simulink model "EV"  (R2023a)
settings: Solver=ode4  StartTime=0.0  StopTime=10  FixedStep=Ts  RelTol=1e-3  EnableMultiTasking=on
PostLoadFcn:
  | Ts=1/1000000;L=1.8e-3;w=2*pi*60;C=20e-6;
InitFcn:
  | Ts=1/1000000;L=1.8e-3;w=2*pi*60;C=20e-6;
undefined symbols (not defined in the file): DiscIntNeverNeededParam
libraries: simulink x13, spsSeriesRLCBranchLib x9, spsIGBTDiodeLib x6, spsGroundLib x5, spsVoltageMeasurementLib x4, spsCurrentMeasurementLib x3, spsDCVoltageSourceLib x1, eePwmGeneratorTwoLevel x1, spspowerguiLib x1
Description:
  | Model of a simple control system for use iin training.
settings Model: Creator=Paul Baracos  LastModifiedBy=Julian
settings SolverCC: AlgebraicLoopSolver=TrustRegion
settings DataIOCC: LimitDataPoints=on  SaveFormat=Array  SignalLoggingSaveFormat=ModelDataLogs  SaveOutput=off  SaveTime=off  ReturnWorkspaceOutputs=off  SignalLoggingName=sigsOut
settings OptimizationCC: BlockReduction=off  BooleanDataType=off  OptimizeBlockIOStorage=off  BufferReuse=off  ReuseModelBlockBuffer=off  GlobalBufferReuse=off  ExpressionFolding=off  LocalBlockOutputs=off  InitFltsAndDblsToZero=on  LifeSpan=inf
settings DebuggingCC: SaveWithParameterizedLinksMsg=none  UnderspecifiedInitializationDetection=Classic  MergeDetectMultiDrivingBlocksExec=none  SignalResolutionControl=TryResolveAllWithWarning  MultiTaskDSMMsg=warning  MultiTaskCondExecSysMsg=none  FcnCallInpInsideContextMsg=warning  UnconnectedInputMsg=warning  UnconnectedOutputMsg=warning  UnconnectedLineMsg=warning  SFUnexpectedBacktrackingDiag=warning  SFNoUnconditionalDefaultTransitionDiag=warning  SFExecutionAtInitializationDiag=none  ArithmeticOperatorsInVariantConditions=warning
settings HardwareCC: ProdBitPerPointer=32  ProdBitPerSizeT=32  ProdBitPerPtrDiffT=32  ProdLargestAtomicFloat=None  ProdIntDivRoundTo=Undefined  ProdEndianess=Unspecified  ProdWordSize=32  ProdHWDeviceType=32-bit Generic  TargetUnknown=on
settings ModelReferenceCC: EnableRefExpFcnMdlSchedulingChecks=on  PropagateSignalLabelsOutOfModel=off
settings SFSimCC: SimUseLocalCustomCode=off  CustomCodeUndefinedFunction=UseInterfaceOnly
settings RTWCC: RTWUseLocalCustomCode=off
settings CodeAppCC: StateflowObjectComments=on
settings GRTTargetCC: TargetFcnLib=ansi_tfl_tmw.mat  TargetLangStandard=C89/C90 (ANSI)  CombineOutputUpdateFcns=off  GRTInterface=on
settings ConfigComp: CovMetricSettings=dw  CovSaveCumulativeToWorkspaceVar=on  CovSaveSingleToWorkspaceVar=on  CovExternalEMLEnable=off
settings SimscapeCC: SimscapeNormalizeSystem=off

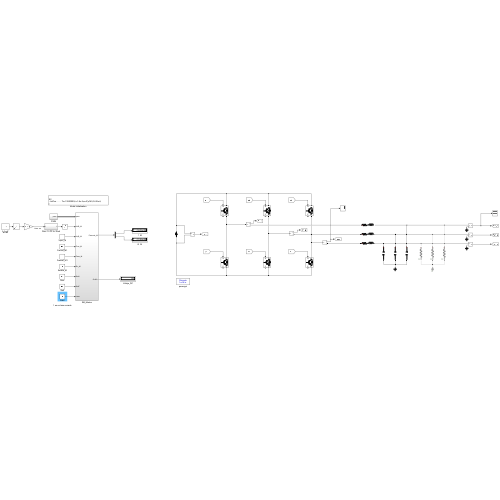
[thumbnail: Simulink's stored preview of the top-level diagram]
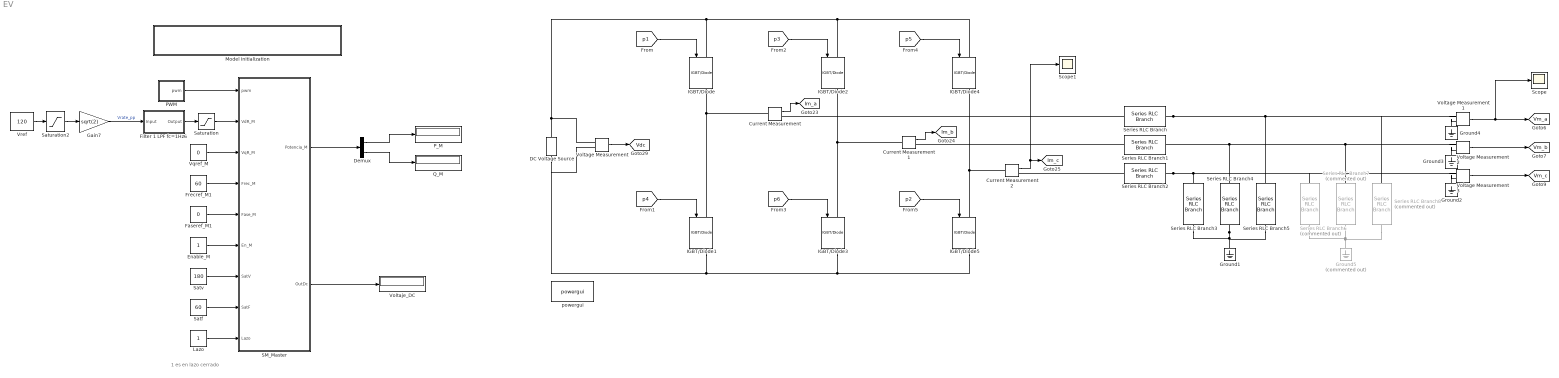
== system EV ==
  note: 1 es en lazo cerrado
  Current Measurement : spsCurrentMeasurementLib/Current Measurement  PhasorSimulation=off  OutputType=Complex  PSBequivalent=0
  Current Measurement1 : spsCurrentMeasurementLib/Current Measurement  PhasorSimulation=off  OutputType=Complex  PSBequivalent=0
  Current Measurement2 : spsCurrentMeasurementLib/Current Measurement  PhasorSimulation=off  OutputType=Complex  PSBequivalent=0
  DC Voltage Source : spsDCVoltageSourceLib/DC Voltage Source  Amplitude=500  Measurements=None
  Demux : Demux  Outputs=2
  Enable_M : Constant
  Faseref_M1 : Constant  Value=0
  Filter 1 LPF fc=1Hz6 : Subsystem  Tag=FilterWizardSubSystem
      settings: ErrorFcn=dspFilterRealizedInBasicElemsAlgLoopErrFcnCallback
  Frecref_M1 : Constant  Value=60
  Gain7 : Gain  Gain=sqrt(2)  SaturateOnIntegerOverflow=on  OutDataTypeStr=Inherit: Same as input  ParamDataTypeStr=Inherit: Same as input
  Ground{1..4} (4 alike) : spsGroundLib/Ground  LConnTagsString=a
  Ground5 : spsGroundLib/Ground  Commented=on  LConnTagsString=a
  IGBT/Diode{,1..5} (6 alike) : spsIGBTDiodeLib/IGBT//Diode  Ron=1e-3  Rs=1e5  Cs=inf  Measurements=on
  Lazo : Constant
  Model Initialization : Subsystem  AncestorBlock=artemis/Tools /Misc/Model Initialization  mask(Model Functions){InitFcnX=Ts=1/1000000;L=1.8e-3;w=2*pi*60;C=20e-6;, prel=off, posl=on, inif=on, strf=off}
      mask prompts: InitFcnX "Initialisation"; prel "Preload Function"; posl "PostLoad Function"; inif "InitFcn"; strf "StartFcn"
      mask init:
      | currentBlock = gcb;
      | root = bdroot(currentBlock);
      | 
      | if ~strcmp(get_param(root,'BlockDiagramType'),'library')
      |     if prel==1
      |         set_param(root, 'PreLoadFcn', InitFcnX);
      |     else
      |         set_param(root, 'PreLoadFcn', '');
      |     end
      |     if inif==1
      |         set_param(root, 'InitFcn', InitFcnX);
      |     else
      |         set_param(root, 'InitFcn', '');
      |     end
      |     if strf==1
      |         set_param(root, 'StartFcn', InitFcnX);
      |     else
      |         set_param(root, 'StartFcn', '');
      |     end
      |     if posl==1
      |         set_param(root, 'PostLoadFcn', InitFcnX);
      |     else
      |         set_param(root, 'PostLoadFcn', '');
      |     end
      | end
      | 
      | pos = get_param(currentBlock, 'Position');
      | width = pos(3) - pos(1); height = pos(4) - pos(2);
      | txt = [ upper(root) '\n' '- InitFcn. . . . . '  get_param(root, 'InitFcn') ];
      settings: LibrarySourceBlock=artemis/Tools /Misc/Model Initialization  CopyFcn=set_param(gcb,'LinkStatus','inactive')
      mask Display: text(5, height*0.5, txt, 'horizontalAlignment', 'left', 'verticalAlignment', 'middle') ;
  PWM : Subsystem
  P_M : Display
  Q_M : Display
  SM_Master : Subsystem
  Satf : Constant  Value=60
  Saturation : Saturate  UpperLimit=180  LowerLimit=0
  Saturation2 : Saturate  UpperLimit=230  LowerLimit=0
  Satv : Constant  Value=180
  Scope : Scope
  Scope1 : Scope
  Series RLC Branch : spsSeriesRLCBranchLib/Series RLC Branch  LConnTagsString=__new0  RConnTagsString=__new0  BranchType=RL  Resistance=0.000001  Inductance=L  SetiL0=off  InitialCurrent=0  Capacitance=1e-6  Setx0=off  InitialVoltage=0  Measurements=None
  Series RLC Branch1 : spsSeriesRLCBranchLib/Series RLC Branch  LConnTagsString=__new0  RConnTagsString=__new0  BranchType=RL  Resistance=0.000001  Inductance=L  SetiL0=off  InitialCurrent=0  Capacitance=1e-6  Setx0=off  InitialVoltage=0  Measurements=None
  Series RLC Branch2 : spsSeriesRLCBranchLib/Series RLC Branch  LConnTagsString=__new0  RConnTagsString=__new0  BranchType=RL  Resistance=0.000001  Inductance=L  SetiL0=off  InitialCurrent=0  Capacitance=1e-6  Setx0=off  InitialVoltage=0  Measurements=None
  Series RLC Branch3 : spsSeriesRLCBranchLib/Series RLC Branch  LConnTagsString=__new0  RConnTagsString=__new0  BranchType=C  Resistance=0.1  Inductance=L  SetiL0=off  InitialCurrent=0  Capacitance=C  Setx0=off  InitialVoltage=0  Measurements=None
  Series RLC Branch4 : spsSeriesRLCBranchLib/Series RLC Branch  LConnTagsString=__new0  RConnTagsString=__new0  BranchType=C  Resistance=0.1  Inductance=L  SetiL0=off  InitialCurrent=0  Capacitance=C  Setx0=off  InitialVoltage=0  Measurements=None
  Series RLC Branch5 : spsSeriesRLCBranchLib/Series RLC Branch  LConnTagsString=__new0  RConnTagsString=__new0  BranchType=C  Resistance=0.1  Inductance=L  SetiL0=off  InitialCurrent=0  Capacitance=C  Setx0=off  InitialVoltage=0  Measurements=None
  Series RLC Branch6 : spsSeriesRLCBranchLib/Series RLC Branch  Commented=on  LConnTagsString=__new0  RConnTagsString=__new0  BranchType=R  Resistance=1  Inductance=L  SetiL0=off  InitialCurrent=0  Capacitance=C  Setx0=off  InitialVoltage=0  Measurements=None
  Series RLC Branch7 : spsSeriesRLCBranchLib/Series RLC Branch  Commented=on  LConnTagsString=__new0  RConnTagsString=__new0  BranchType=R  Resistance=1  Inductance=L  SetiL0=off  InitialCurrent=0  Capacitance=100  Setx0=off  InitialVoltage=0  Measurements=None
  Series RLC Branch8 : spsSeriesRLCBranchLib/Series RLC Branch  Commented=on  LConnTagsString=__new0  RConnTagsString=__new0  BranchType=R  Resistance=1  Inductance=L  SetiL0=off  InitialCurrent=0  Capacitance=C  Setx0=off  InitialVoltage=0  Measurements=None
  Voltage Measurement{,1..3} (4 alike) : spsVoltageMeasurementLib/Voltage Measurement  PhasorSimulation=off  OutputType=Complex  PSBequivalent=0
  Voltaje_DC : Display
  Vqref_M : Constant  Value=0
  Vref : Constant  Value=120
  powergui : spspowerguiLib/powergui  Priority=1  SimulationMode=Discrete  SampleTime=Ts  frequency=60  Iterations=50  frequencyindice=0  Pbase=100e6  ErrMax=1e-4  UnitsV=kV  UnitsW=MW  buscounter=0  FunctionMessages=off  echomessages=off  EnableUseOfTLC=off  CurrentSourceSwitches=off  DisableSnubberDevices=off  DisableRonSwitches=off  DisableVfSwitches=off  DisplayEquations=off  AutomaticDiscreteSolvers=off  SolverType=Tustin/Backward Euler (TBE)  Interpol=off  ExternalGateDelay=off  methode=off  Ts=100  x0status=blocks  SPID=on  SwTol=0  HookPort=off  NonlinearTolerance=1e-4  nMaxIteration=100  ContinueOnMaxIteration=off  RestoreLinks=warning  ResistiveCurrentMeasurement=off  Frange=[0:2:500]  Ylog=off  Xlog=on  ShowGrid=off  save=off  variable=ZData  structure=0  ZoomFFT=off  StartTime=0.0  cycles=1  DisplayStyle=1  fundamental=60  FreqAxis=off  MaxFrequency=1000  frequencyindicesteady=1  RmsSteady=1  display=off
  tag scope: Im_a=global, Im_b=global, Im_c=global, Vdc=global, Vm_a=global, Vm_b=global, Vm_c=global
  wires:
  Filter 1 LPF fc=1Hz6/1(Output) -> Saturation/1
  Saturation2/1 -> Gain7/1
  Gain7/1 -> Filter 1 LPF fc=1Hz6/1(Input)  "Vrate_pp"
  Vref/1 -> Saturation2/1
  Demux/1 -> P_M/1
  Demux/2 -> Q_M/1
  SM_Master/1(Potencia_M) -> Demux/1
  [p4] -> IGBT/Diode1/1
  [p2] -> IGBT/Diode5/1
  [p5] -> IGBT/Diode4/1
  [p3] -> IGBT/Diode2/1
  [p1] -> IGBT/Diode/1
  [p6] -> IGBT/Diode3/1
  Voltage Measurement/1 -> [Vdc]
  Current Measurement/1 -> [Im_a]
  Current Measurement1/1 -> [Im_b]
  Current Measurement2/1 -> Scope1/1, [Im_c]
  Voltage Measurement3/1 -> [Vm_c]
  Voltage Measurement2/1 -> [Vm_b]
  Voltage Measurement1/1 -> Scope/1, [Vm_a]
  Saturation/1 -> SM_Master/2(VdR_M)
  SM_Master/2(OutDc) -> Voltaje_DC/1
  Vqref_M/1 -> SM_Master/3(VqR_M)
  Frecref_M1/1 -> SM_Master/4(Frec_M)
  Faseref_M1/1 -> SM_Master/5(Fase_M)
  Enable_M/1 -> SM_Master/6(En_M)
  Satv/1 -> SM_Master/7(SatV)
  Satf/1 -> SM_Master/8(SatF)
  Lazo/1 -> SM_Master/9(Lazo)
  PWM/1("pwm ") -> SM_Master/1("pwm ")
  connections:
  IGBT/Diode5/LConn1 -- Current Measurement2/LConn1 -- IGBT/Diode4/RConn1
  IGBT/Diode3/LConn1 -- Current Measurement1/LConn1 -- IGBT/Diode2/RConn1
  IGBT/Diode3/RConn1 -- IGBT/Diode5/RConn1 -- Voltage Measurement/LConn2 -- DC Voltage Source/LConn1 -- IGBT/Diode1/RConn1
  IGBT/Diode2/LConn1 -- IGBT/Diode4/LConn1 -- IGBT/Diode/LConn1 -- DC Voltage Source/RConn1 -- Voltage Measurement/LConn1
  IGBT/Diode1/LConn1 -- Current Measurement/LConn1 -- IGBT/Diode/RConn1
  Series RLC Branch2/LConn1 -- Current Measurement2/RConn1
  Series RLC Branch1/LConn1 -- Current Measurement1/RConn1
  Series RLC Branch/LConn1 -- Current Measurement/RConn1
  Voltage Measurement2/LConn1 -- Series RLC Branch7/LConn1 -- Series RLC Branch4/LConn1 -- Series RLC Branch1/RConn1
  Series RLC Branch/RConn1 -- Series RLC Branch8/LConn1 -- Voltage Measurement1/LConn1 -- Series RLC Branch5/LConn1
  Series RLC Branch4/RConn1 -- Series RLC Branch3/RConn1 -- Ground1/LConn1 -- Series RLC Branch5/RConn1
  Series RLC Branch2/RConn1 -- Series RLC Branch6/LConn1 -- Voltage Measurement3/LConn1 -- Series RLC Branch3/LConn1
  Ground4/LConn1 -- Voltage Measurement1/LConn2
  Ground3/LConn1 -- Voltage Measurement2/LConn2
  Ground2/LConn1 -- Voltage Measurement3/LConn2
  Series RLC Branch8/RConn1 -- Ground5/LConn1 -- Series RLC Branch6/RConn1 -- Series RLC Branch7/RConn1

== system EV/Filter 1 LPF fc=1Hz6 ==
  Input : Inport
  Delay11 : Delay  DelayLength=1
  SumA21 : Sum  Inputs=|+-  RndMeth=Nearest  SaturateOnIntegerOverflow=on  OutDataTypeStr=Inherit: Same as first input
  SumB21 : Sum  Inputs=|++  RndMeth=Nearest  SaturateOnIntegerOverflow=on  OutDataTypeStr=Inherit: Same as first input
  a(2)(1) : Gain  Gain=-0.99937187877871914  ParamDataTypeStr=float('double')  RndMeth=Nearest  SaturateOnIntegerOverflow=on  OutDataTypeStr=Inherit: Same as input
  s(1) : Gain  Gain=0.00031406061064044236  ParamDataTypeStr=float('double')  RndMeth=Nearest  SaturateOnIntegerOverflow=on  OutDataTypeStr=Inherit: Same as input
  Output : Outport
  wires:
  Delay11/1 -> SumB21/2, a(2)(1)/1
  a(2)(1)/1 -> SumA21/2
  SumB21/1 -> Output/1
  SumA21/1 -> Delay11/1, SumB21/1
  s(1)/1 -> SumA21/1
  Input/1 -> s(1)/1

== system EV/Model Initialization ==

== system EV/PWM ==
  A1 : Constant  Value=20
  B1 : Constant  Value=10080
  Bus Creator : BusCreator  Inputs=3
  Bus Creator2 : BusCreator  Inputs=3
  Bus Creator3 : BusCreator  Inputs=2
  "pwm " : Outport
  wires:
  Bus Creator2/1 -> Bus Creator3/1  "FreqPWMOut"
  Bus Creator/1 -> Bus Creator3/2  "DutyPWMOut"
  Bus Creator3/1 -> "pwm "/1  "PWMO_Ch00_07"
  A1/1 -> Bus Creator/2, Bus Creator/3, Bus Creator/1  "DutyCh02"
  B1/1 -> Bus Creator2/1, Bus Creator2/2, Bus Creator2/3  "FreqCh00"

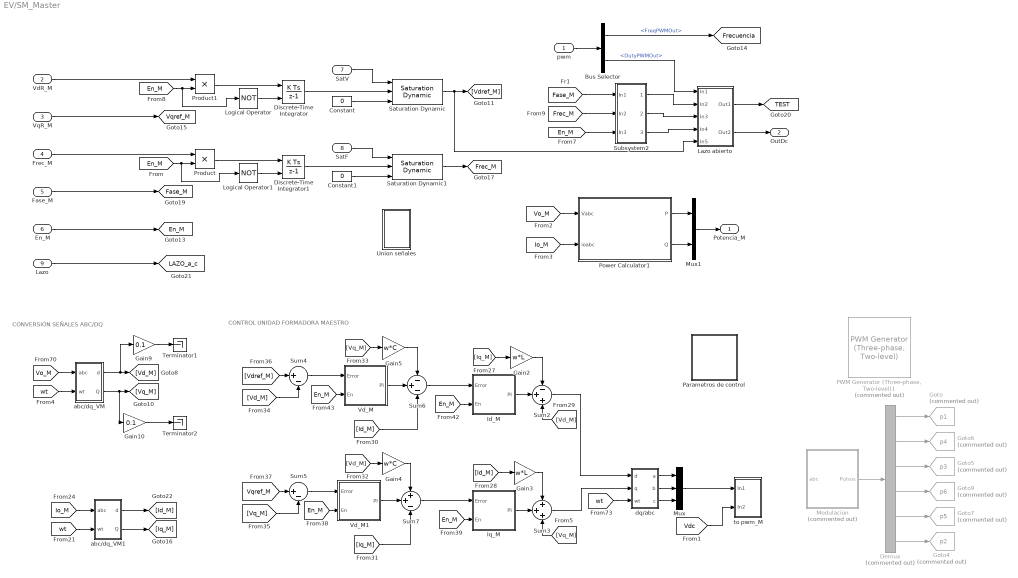
== system EV/SM_Master ==
  note: CONVERSIÓN SEÑALES ABC/DQ
  note: CONTROL UNIDAD FORMADORA MAESTRO
  "pwm " : Inport
  VdR_M : Inport  Port=2
  VqR_M : Inport  Port=3
  Frec_M : Inport  Port=4
  Fase_M : Inport  Port=5
  En_M : Inport  Port=6
  SatV : Inport  Port=7
  SatF : Inport  Port=8
  Lazo : Inport  Port=9
  Bus Selector : BusSelector  OutputSignals=FreqPWMOut,DutyPWMOut
  Constant : Constant  Value=0
  Constant1 : Constant  Value=0
  Demux : Demux  Commented=on  Outputs=6
  Discrete-Time Integrator : DiscreteIntegrator  ExternalReset=level  SampleTime=-1  ICPrevOutput=DiscIntNeverNeededParam  ICPrevScaledInput=DiscIntNeverNeededParam
  Discrete-Time Integrator1 : DiscreteIntegrator  ExternalReset=level  SampleTime=-1  ICPrevOutput=DiscIntNeverNeededParam  ICPrevScaledInput=DiscIntNeverNeededParam
  Gain10 : Gain  Gain=0.1
  Gain2 : Gain  Gain=w*L
  Gain3 : Gain  Gain=w*L
  Gain4 : Gain  Gain=w*C
  Gain5 : Gain  Gain=w*C
  Gain9 : Gain  Gain=0.1
  Goto : Goto  Commented=on  GotoTag=p1  TagVisibility=global
  Goto4 : Goto  Commented=on  GotoTag=p2  TagVisibility=global
  Goto5 : Goto  Commented=on  GotoTag=p3  TagVisibility=global
  Goto6 : Goto  Commented=on  GotoTag=p4  TagVisibility=global
  Goto7 : Goto  Commented=on  GotoTag=p5  TagVisibility=global
  Goto9 : Goto  Commented=on  GotoTag=p6  TagVisibility=global
  Id_M : Subsystem
  Iq_M : Subsystem
  "Lazo abierto " : Subsystem
  Logical Operator : Logic  Operator=NOT  AllPortsSameDT=off  OutDataTypeStr=boolean
  Logical Operator1 : Logic  Operator=NOT  AllPortsSameDT=off  OutDataTypeStr=boolean
  Modulacion : Subsystem  Commented=on
  Mux : Mux  Inputs=3
  Mux1 : Mux  Inputs=2
  "PWM Generator (Three-phase, Two-level)1" : eePwmGeneratorTwoLevel/PWM Generator (Three-phase, Two-level)  Commented=on  PWMMode=Continuous PWM (CPWM)  CPWMMode=SPWM: sinusoidal PWM  DPWMMode=60 DPWM: 60 degree discontinuous PWM  fsw=10000  Ts=Ts
  Parametros de control : Subsystem
  Power Calculator1 : Subsystem
  Product : Product
  Product1 : Product
  Saturation Dynamic : simulink/Discontinuities/Saturation Dynamic  OutMin=[]  OutMax=[]  OutDataTypeStr=Inherit: Same as second input  OutDataType=fixdt(1, 16)  OutScaling=2^-10  DoSatur=off
  Saturation Dynamic1 : simulink/Discontinuities/Saturation Dynamic  OutMin=[]  OutMax=[]  OutDataTypeStr=Inherit: Same as second input  OutDataType=fixdt(1, 16)  OutScaling=2^-10  DoSatur=off
  Subsystem2 : Subsystem
  Sum2 : Sum  Inputs=-++
  Sum3 : Sum  Inputs=+++
  Sum4 : Sum  Inputs=|+-
  Sum5 : Sum  Inputs=|+-
  Sum6 : Sum  Inputs=-+-
  Sum7 : Sum  Inputs=++-
  Terminator1 : Terminator
  Terminator2 : Terminator
  "Union señales " : Subsystem
  Vd_M : Subsystem
  Vd_M1 : Subsystem
  abc/dq_VM : Subsystem
  abc/dq_VM1 : Subsystem
  dq/abc : Subsystem
  to pwm_M : Subsystem
  Potencia_M : Outport
  OutDc : Outport  Port=2
  tag scope: En_M=global, Fase_M=global, Frec_M=global, Frecuencia=global, LAZO_a_c=global, TEST=global, Vqref_M=global
  wires:
  [Vo_M] -> abc/dq_VM/1(abc)
  abc/dq_VM1/1(d) -> [Id_M]
  [Io_M] -> abc/dq_VM1/1(abc)
  abc/dq_VM/2(Q) -> Gain10/1, [Vq_M]
  [wt] -> abc/dq_VM1/2(wt)
  [wt] -> abc/dq_VM/2(wt)
  abc/dq_VM1/2(Q) -> [Iq_M]
  abc/dq_VM/1(d) -> Gain9/1, [Vd_M]
  Gain5/1 -> Sum6/1
  Gain3/1 -> Sum3/1
  [Id_M] -> Gain3/1
  [Vdref_M] -> Sum4/1
  [Vq_M] -> Sum3/3
  Sum7/1 -> Iq_M/1(Error)
  [Id_M] -> Sum6/3
  [Vd_M] -> Gain4/1
  [En_M] -> Vd_M1/2(En)
  [Vq_M] -> Sum5/2
  Sum2/1 -> dq/abc/1(d)
  [En_M] -> Vd_M/2(En)
  dq/abc/3(c) -> Mux/3
  [Iq_M] -> Sum7/3
  [En_M] -> Iq_M/2(En)
  Gain2/1 -> Sum2/1
  [Vq_M] -> Gain5/1
  dq/abc/2(b) -> Mux/2
  dq/abc/1(a) -> Mux/1
  [wt] -> dq/abc/3(wt)
  Gain4/1 -> Sum7/1
  Sum3/1 -> dq/abc/2(q)
  [Vd_M] -> Sum4/2
  Sum5/1 -> Vd_M1/1(Error)
  Id_M/1(PI) -> Sum2/2
  Sum6/1 -> Id_M/1(Error)
  [Vd_M] -> Sum2/3
  Sum4/1 -> Vd_M/1(Error)
  [Iq_M] -> Gain2/1
  Vd_M/1(PI) -> Sum6/2
  Iq_M/1(PI) -> Sum3/2
  [En_M] -> Id_M/2(En)
  [Vqref_M] -> Sum5/1
  Vd_M1/1(PI) -> Sum7/2
  [Vdc] -> to pwm_M/2(In2)
  Gain9/1 -> Terminator1/1
  [Vo_M] -> Power Calculator1/1(Vabc)
  [Io_M] -> Power Calculator1/2(ioabc)
  Power Calculator1/2("Q ") -> Mux1/2
  Power Calculator1/1(P) -> Mux1/1
  Mux1/1 -> Potencia_M/1
  Gain10/1 -> Terminator2/1
  Mux/1 -> to pwm_M/1(In1)
  Demux/1 -> Goto/1
  Demux/2 -> Goto6/1
  Demux/3 -> Goto5/1
  Demux/4 -> Goto9/1
  Demux/5 -> Goto7/1
  Demux/6 -> Goto4/1
  Modulacion/1(Pulsos) -> Demux/1
  Bus Selector/1 -> [Frecuencia]  "<FreqPWMOut>"
  [Fase_M] -> Subsystem2/1(In1)
  Subsystem2/1(Out1) -> "Lazo abierto "/2(In2)
  Constant/1 -> Saturation Dynamic/3
  Discrete-Time Integrator/1 -> Saturation Dynamic/2
  "Lazo abierto "/2(Out2) -> OutDc/1
  Saturation Dynamic/1 -> "Lazo abierto "/5(In5), [Vdref_M]
  "Lazo abierto "/1(Out1) -> [TEST]
  Logical Operator1/1 -> Discrete-Time Integrator1/2
  Subsystem2/2(Out2) -> "Lazo abierto "/3(In3)
  Logical Operator/1 -> Discrete-Time Integrator/2
  [En_M] -> Logical Operator1/1, Product/2
  "pwm "/1 -> Bus Selector/1
  Saturation Dynamic1/1 -> [Frec_M]
  Subsystem2/3(Out3) -> "Lazo abierto "/4(In4)
  [En_M] -> Logical Operator/1, Product1/2
  Product1/1 -> Discrete-Time Integrator/1
  Discrete-Time Integrator1/1 -> Saturation Dynamic1/2
  Constant1/1 -> Saturation Dynamic1/3
  [En_M] -> Subsystem2/3(In3)
  Product/1 -> Discrete-Time Integrator1/1
  Bus Selector/2 -> "Lazo abierto "/1(In1)  "<DutyPWMOut>"
  [Frec_M] -> Subsystem2/2(In2)
  Lazo/1 -> [LAZO_a_c]
  SatF/1 -> Saturation Dynamic1/1
  SatV/1 -> Saturation Dynamic/1
  En_M/1 -> [En_M]
  Fase_M/1 -> [Fase_M]
  VqR_M/1 -> [Vqref_M]
  Frec_M/1 -> Product/1
  VdR_M/1 -> Product1/1

== system EV/SM_Master/Id_M ==
  Error : Inport
  En : Inport  Port=2
  Constant2 : Constant  Value=0
  FF Int : DiscreteIntegrator  ExternalReset=level  InitialConditionSource=external  InitialCondition=4  SampleTime=Ts  ICPrevOutput=DiscIntNeverNeededParam  ICPrevScaledInput=DiscIntNeverNeededParam
  Logical Operator : Logic  Operator=NOT  AllPortsSameDT=off  OutDataTypeStr=boolean
  Subsystem : Subsystem
  Subsystem1 : Subsystem
  Sum3 : Sum  OutDataTypeStr=Inherit: Same as first input
  PI : Outport
  wires:
  Subsystem/1(X*Y) -> Sum3/1
  Error/1 -> Subsystem1/1(X), Subsystem/2(Y)
  [Ki_IM] -> Subsystem1/2(Y)
  [Kp_IM] -> Subsystem/1(X)
  Sum3/1 -> PI/1
  En/1 -> Logical Operator/1, Subsystem1/3(En), Subsystem/3(En)
  Logical Operator/1 -> FF Int/2
  Constant2/1 -> FF Int/3
  Subsystem1/1(X*Y) -> FF Int/1
  FF Int/1 -> Sum3/2

== system EV/SM_Master/Iq_M ==
  Error : Inport
  En : Inport  Port=2
  Constant2 : Constant  Value=0
  FF Int : DiscreteIntegrator  ExternalReset=level  InitialConditionSource=external  InitialCondition=4  SampleTime=Ts  ICPrevOutput=DiscIntNeverNeededParam  ICPrevScaledInput=DiscIntNeverNeededParam
  Logical Operator : Logic  Operator=NOT  AllPortsSameDT=off  OutDataTypeStr=boolean
  Subsystem : Subsystem
  Subsystem1 : Subsystem
  Sum3 : Sum  OutDataTypeStr=Inherit: Same as first input
  PI : Outport
  wires:
  Subsystem/1(X*Y) -> Sum3/1
  Error/1 -> Subsystem1/1(X), Subsystem/2(Y)
  [Ki_IM] -> Subsystem1/2(Y)
  [Kp_IM] -> Subsystem/1(X)
  Sum3/1 -> PI/1
  En/1 -> Logical Operator/1, Subsystem1/3(En), Subsystem/3(En)
  Logical Operator/1 -> FF Int/2
  Constant2/1 -> FF Int/3
  Subsystem1/1(X*Y) -> FF Int/1
  FF Int/1 -> Sum3/2

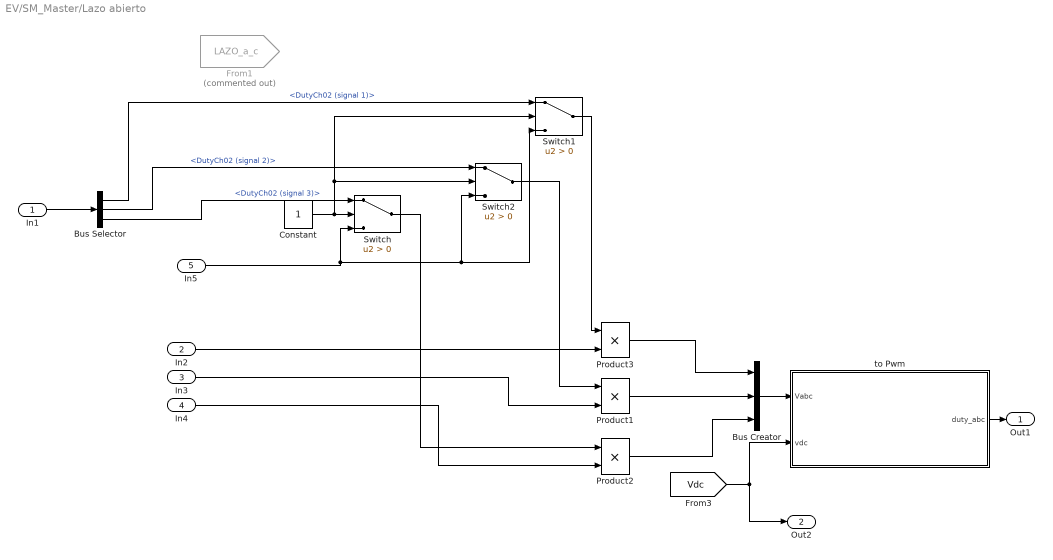
== system EV/SM_Master/Lazo abierto  ==
  In1 : Inport
  In2 : Inport  Port=2
  In3 : Inport  Port=3
  In4 : Inport  Port=4
  In5 : Inport  Port=5
  Bus Creator : BusCreator  Inputs=3
  Bus Selector : BusSelector  OutputSignals=DutyCh02 (signal 1),DutyCh02 (signal 2),DutyCh02 (signal 3)
  Constant : Constant
  From1 : From  Commented=on  GotoTag=LAZO_a_c  TagVisibility=global
  Product1 : Product  RndMeth=Zero
  Product2 : Product  RndMeth=Zero
  Product3 : Product  RndMeth=Zero
  Switch : Switch  Criteria=u2 > Threshold  SaturateOnIntegerOverflow=off  InputSameDT=off
  Switch1 : Switch  Criteria=u2 > Threshold  SaturateOnIntegerOverflow=off  InputSameDT=off
  Switch2 : Switch  Criteria=u2 > Threshold  SaturateOnIntegerOverflow=off  InputSameDT=off
  to Pwm : Subsystem
      mask Display:
      | disp('Modulation');
      | port_label('input', 1, 'Vpwm');
      | port_label('input', 2, 'Vdc');
      | port_label('output', 1, 'duty');
  Out1 : Outport
  Out2 : Outport  Port=2
  wires:
  In3/1 -> Product1/2
  In4/1 -> Product2/2
  In2/1 -> Product3/2
  [Vdc] -> Out2/1, to Pwm/2(vdc)
  Product3/1 -> Bus Creator/1
  Product1/1 -> Bus Creator/2
  Product2/1 -> Bus Creator/3
  to Pwm/1(duty_abc) -> Out1/1
  Bus Creator/1 -> to Pwm/1(Vabc)
  In1/1 -> Bus Selector/1
  Bus Selector/3 -> Switch/1  "<DutyCh02 (signal 3)>"
  In5/1 -> Switch1/3, Switch2/3, Switch/3
  Constant/1 -> Switch1/2, Switch2/2, Switch/2
  Switch/1 -> Product2/1
  Switch2/1 -> Product1/1
  Bus Selector/2 -> Switch2/1  "<DutyCh02 (signal 2)>"
  Bus Selector/1 -> Switch1/1  "<DutyCh02 (signal 1)>"
  Switch1/1 -> Product3/1

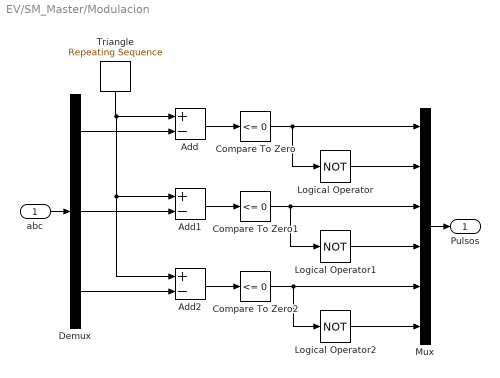
== system EV/SM_Master/Modulacion ==
  abc : Inport
  Add : Sum  Inputs=+-
  Add1 : Sum  Inputs=+-
  Add2 : Sum  Inputs=+-
  Compare To Zero : simulink/Logic and Bit Operations/Compare To Zero  relop=<=  OutDataTypeStr=boolean  ZeroCross=off
  Compare To Zero1 : simulink/Logic and Bit Operations/Compare To Zero  relop=<=  OutDataTypeStr=boolean  ZeroCross=off
  Compare To Zero2 : simulink/Logic and Bit Operations/Compare To Zero  relop=<=  OutDataTypeStr=boolean  ZeroCross=off
  Demux : Demux  Outputs=3
  Logical Operator : Logic  Operator=NOT  AllPortsSameDT=off  OutDataTypeStr=boolean
  Logical Operator1 : Logic  Operator=NOT  AllPortsSameDT=off  OutDataTypeStr=boolean
  Logical Operator2 : Logic  Operator=NOT  AllPortsSameDT=off  OutDataTypeStr=boolean
  Mux : Mux  Inputs=6
  Triangle : simulink/Sources/Repeating Sequence  rep_seq_t=[0 2/Fc/4 3/Fc/4 1/Fc]  rep_seq_y=[-1 1 0 -1]  mask(Repeating table){Fc=100000}
      mask help: (Fc) Frequncia de portadora
      mask DialogControl Fc Tooltip: Fc
  Pulsos : Outport
  wires:
  Add/1 -> Compare To Zero/1
  Add1/1 -> Compare To Zero1/1
  Triangle/1 -> Add/1, Add1/1, Add2/1
  abc/1 -> Demux/1
  Add2/1 -> Compare To Zero2/1
  Demux/1 -> Add/2
  Demux/3 -> Add2/2
  Demux/2 -> Add1/2
  Mux/1 -> Pulsos/1
  Compare To Zero/1 -> Mux/1, Logical Operator/1
  Logical Operator/1 -> Mux/2
  Compare To Zero1/1 -> Mux/3, Logical Operator1/1
  Logical Operator1/1 -> Mux/4
  Compare To Zero2/1 -> Mux/5, Logical Operator2/1
  Logical Operator2/1 -> Mux/6

== system EV/SM_Master/Parametros de control ==
  Constant : Constant  Value=0.0655
  Constant1 : Constant  Value=22.739
  Constant2 : Constant  Value=20
  Constant3 : Constant  Value=50
  tag scope: Ki_IM=global, Ki_VM=global, Kp_IM=global, Kp_VM=global
  wires:
  Constant3/1 -> [Ki_IM]
  Constant1/1 -> [Ki_VM]
  Constant2/1 -> [Kp_IM]
  Constant/1 -> [Kp_VM]

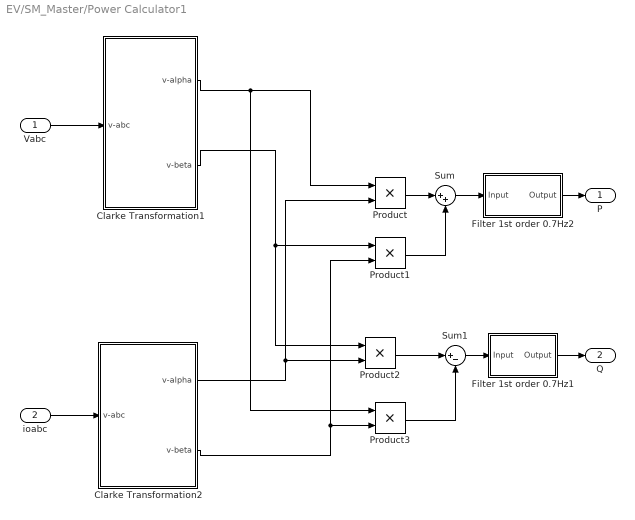
== system EV/SM_Master/Power Calculator1 ==
  Vabc : Inport
  ioabc : Inport  Port=2
  Clarke Transformation1 : Subsystem
  Clarke Transformation2 : Subsystem
  Filter 1st order 0.7Hz1 : Subsystem  Tag=FilterWizardSubSystem
      settings: ErrorFcn=dspFilterRealizedInBasicElemsAlgLoopErrFcnCallback
  Filter 1st order 0.7Hz2 : Subsystem  Tag=FilterWizardSubSystem
      settings: ErrorFcn=dspFilterRealizedInBasicElemsAlgLoopErrFcnCallback
  Product{,1..3} (4 alike) : Product  RndMeth=Zero
  Sum : Sum  Inputs=|++
  Sum1 : Sum  Inputs=|+-
  P : Outport
  "Q " : Outport  Port=2
  wires:
  Vabc/1 -> Clarke Transformation1/1(v-abc)
  ioabc/1 -> Clarke Transformation2/1(v-abc)
  Product/1 -> Sum/1
  Product1/1 -> Sum/2
  Product2/1 -> Sum1/1
  Product3/1 -> Sum1/2
  Sum/1 -> Filter 1st order 0.7Hz2/1(Input)
  Sum1/1 -> Filter 1st order 0.7Hz1/1(Input)
  Clarke Transformation1/1(v-alpha) -> Product3/1, Product/1
  Clarke Transformation1/2(v-beta) -> Product1/1, Product2/1
  Clarke Transformation2/1(v-alpha) -> Product2/2, Product/2
  Clarke Transformation2/2(v-beta) -> Product3/2, Product1/2
  Filter 1st order 0.7Hz1/1(Output) -> "Q "/1
  Filter 1st order 0.7Hz2/1(Output) -> P/1

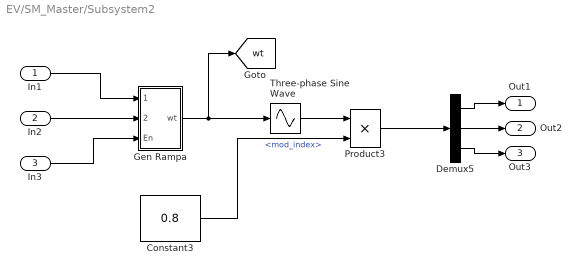
== system EV/SM_Master/Subsystem2 ==
  In1 : Inport
  In2 : Inport  Port=2
  In3 : Inport  Port=3
  Constant3 : Constant  Value=0.8
  Demux5 : Demux  Outputs=3
  Gen Rampa : Subsystem
  Product3 : Product  RndMeth=Zero
  Three-phase Sine Wave : Sin  TimeSource=Use external signal  Phase=[0 -2*pi/3 2*pi/3]
  Out1 : Outport
  Out2 : Outport  Port=2
  Out3 : Outport  Port=3
  tag scope: wt=global
  wires:
  Demux5/1 -> Out1/1
  Product3/1 -> Demux5/1
  Demux5/2 -> Out2/1
  Three-phase Sine Wave/1 -> Product3/1
  Constant3/1 -> Product3/2  "<mod_index>"
  Demux5/3 -> Out3/1
  Gen Rampa/1("wt ") -> [wt], Three-phase Sine Wave/1
  In3/1 -> Gen Rampa/3(En)
  In2/1 -> Gen Rampa/2(Frec)
  In1/1 -> Gen Rampa/1(Fase)

== system EV/SM_Master/Union señales  ==
  Mux1 : Mux  Inputs=3
  Mux5 : Mux  Inputs=3
  tag scope: Io_M=global, Vo_M=global
  wires:
  [Im_b] -> Mux5/2
  Mux5/1 -> [Io_M]
  [Im_c] -> Mux5/3
  [Vm_a] -> Mux1/1
  [Vm_c] -> Mux1/3
  [Im_a] -> Mux5/1
  Mux1/1 -> [Vo_M]
  [Vm_b] -> Mux1/2

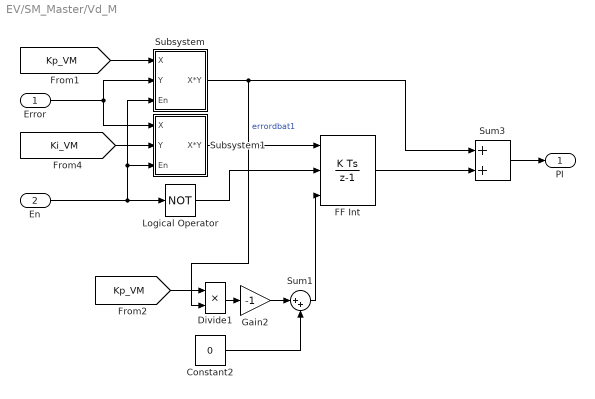
== system EV/SM_Master/Vd_M ==
  Error : Inport
  En : Inport  Port=2
  Constant2 : Constant  Value=0
  Divide1 : Product  Inputs=**  OutDataTypeStr=Inherit: Same as first input
  FF Int : DiscreteIntegrator  ExternalReset=level  InitialConditionSource=external  InitialCondition=4  SampleTime=Ts  ICPrevOutput=DiscIntNeverNeededParam  ICPrevScaledInput=DiscIntNeverNeededParam
  Gain2 : Gain  Gain=-1
  Logical Operator : Logic  Operator=NOT  AllPortsSameDT=off  OutDataTypeStr=boolean
  Subsystem : Subsystem
  Subsystem1 : Subsystem
  Sum1 : Sum  Inputs=|++
  Sum3 : Sum  OutDataTypeStr=Inherit: Same as first input
  PI : Outport
  wires:
  Error/1 -> Subsystem1/1(X), Subsystem/2(Y)
  [Ki_VM] -> Subsystem1/2(Y)
  [Kp_VM] -> Subsystem/1(X)
  Sum3/1 -> PI/1
  En/1 -> Logical Operator/1, Subsystem1/3(En), Subsystem/3(En)
  Logical Operator/1 -> FF Int/2
  Gain2/1 -> Sum1/1
  [Kp_VM] -> Divide1/1
  Divide1/1 -> Gain2/1
  Subsystem/1(X*Y) -> Divide1/2, Sum3/1  "errordbat1"
  Sum1/1 -> FF Int/3
  Constant2/1 -> Sum1/2
  Subsystem1/1(X*Y) -> FF Int/1
  FF Int/1 -> Sum3/2

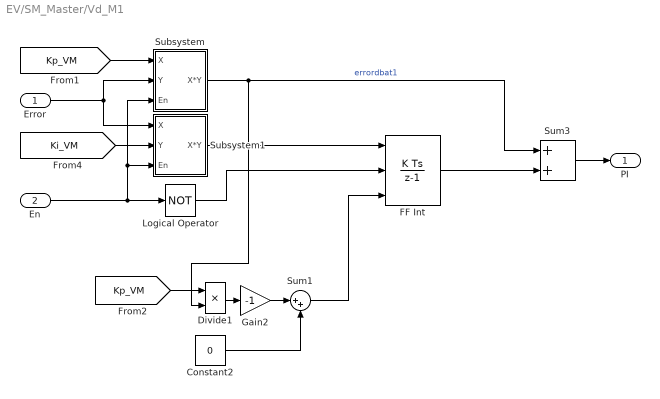
== system EV/SM_Master/Vd_M1 ==
  Error : Inport
  En : Inport  Port=2
  Constant2 : Constant  Value=0
  Divide1 : Product  Inputs=**  OutDataTypeStr=Inherit: Same as first input
  FF Int : DiscreteIntegrator  ExternalReset=level  InitialConditionSource=external  InitialCondition=4  SampleTime=Ts  ICPrevOutput=DiscIntNeverNeededParam  ICPrevScaledInput=DiscIntNeverNeededParam
  Gain2 : Gain  Gain=-1
  Logical Operator : Logic  Operator=NOT  AllPortsSameDT=off  OutDataTypeStr=boolean
  Subsystem : Subsystem
  Subsystem1 : Subsystem
  Sum1 : Sum  Inputs=|++
  Sum3 : Sum  OutDataTypeStr=Inherit: Same as first input
  PI : Outport
  wires:
  Error/1 -> Subsystem1/1(X), Subsystem/2(Y)
  [Ki_VM] -> Subsystem1/2(Y)
  [Kp_VM] -> Subsystem/1(X)
  Sum3/1 -> PI/1
  En/1 -> Logical Operator/1, Subsystem1/3(En), Subsystem/3(En)
  Logical Operator/1 -> FF Int/2
  Gain2/1 -> Sum1/1
  [Kp_VM] -> Divide1/1
  Divide1/1 -> Gain2/1
  Subsystem/1(X*Y) -> Divide1/2, Sum3/1  "errordbat1"
  Sum1/1 -> FF Int/3
  Constant2/1 -> Sum1/2
  Subsystem1/1(X*Y) -> FF Int/1
  FF Int/1 -> Sum3/2

== system EV/SM_Master/abc//dq_VM ==
  abc : Inport
  wt : Inport  Port=2
  Subsystem2 : Subsystem
  abc/alfabeta2 : Subsystem  mask{k=2/3}
  d : Outport
  Q : Outport  Port=2
  wires:
  abc/alfabeta2/1(alfa) -> Subsystem2/1(alfa)
  abc/alfabeta2/2(Beta) -> Subsystem2/2(beta)
  wt/1 -> Subsystem2/3(wt)
  Subsystem2/2(Q) -> Q/1
  abc/1 -> abc/alfabeta2/1(abc)
  Subsystem2/1(d) -> d/1

== system EV/SM_Master/abc//dq_VM1 ==
  abc : Inport
  wt : Inport  Port=2
  Subsystem2 : Subsystem
  abc/alfabeta2 : Subsystem  mask{k=2/3}
  d : Outport
  Q : Outport  Port=2
  wires:
  Subsystem2/1(d) -> d/1
  abc/1 -> abc/alfabeta2/1(abc)
  Subsystem2/2(Q) -> Q/1
  wt/1 -> Subsystem2/3(wt)
  abc/alfabeta2/2(Beta) -> Subsystem2/2(beta)
  abc/alfabeta2/1(alfa) -> Subsystem2/1(alfa)

== system EV/SM_Master/dq//abc ==
  d : Inport
  q : Inport  Port=2
  wt : Inport  Port=3
  Subsystem1 : Subsystem  mask{k=1}
  dq/alfabeta1 : Subsystem
  a : Outport
  b : Outport  Port=2
  c : Outport  Port=3
  wires:
  dq/alfabeta1/1(alfa) -> Subsystem1/1(alfa)
  dq/alfabeta1/2(beta) -> Subsystem1/2(beta)
  wt/1 -> dq/alfabeta1/3(wt)
  d/1 -> dq/alfabeta1/1(d)
  Subsystem1/1(a) -> a/1
  Subsystem1/3(c) -> c/1
  Subsystem1/2(b) -> b/1
  q/1 -> dq/alfabeta1/2(q)

== system EV/SM_Master/to pwm_M ==
  In1 : Inport
  In2 : Inport  Port=2
  Bus Creator2 : BusCreator  Inputs=3
  Demux1 : Demux  Outputs=3
  Salida PWM : Subsystem
  Switch : Switch  Criteria=u2 > Threshold  SaturateOnIntegerOverflow=off  InputSameDT=off
  to Pwm1 : Subsystem
      mask Display:
      | disp('Modulation');
      | port_label('input', 1, 'Vpwm');
      | port_label('input', 2, 'Vdc');
      | port_label('output', 1, 'duty');
  wires:
  In1/1 -> to Pwm1/1(Vabc)
  Demux1/3 -> Bus Creator2/3
  Demux1/1 -> Bus Creator2/1
  In2/1 -> to Pwm1/2(vdc)
  Demux1/2 -> Bus Creator2/2
  Bus Creator2/1 -> Salida PWM/1("ciclo util ")
  [TEST] -> Switch/3
  [LAZO_a_c] -> Switch/2
  Switch/1 -> Demux1/1
  to Pwm1/1(duty_abc) -> Switch/1

== system EV/SM_Master/Id_M/Subsystem ==
  X : Inport
  Y : Inport  Port=2
  En : Inport  Port=3
  Divide2 : Product  Inputs=**  OutDataTypeStr=Inherit: Same as first input
  Divide5 : Product  Inputs=**  OutDataTypeStr=Inherit: Same as first input
  X*Y : Outport
  wires:
  X/1 -> Divide2/1
  En/1 -> Divide5/2
  Divide2/1 -> Divide5/1
  Divide5/1 -> X*Y/1
  Y/1 -> Divide2/2

== system EV/SM_Master/Id_M/Subsystem1 ==
  X : Inport
  Y : Inport  Port=2
  En : Inport  Port=3
  Divide2 : Product  Inputs=**  OutDataTypeStr=Inherit: Same as first input
  Divide5 : Product  Inputs=**  OutDataTypeStr=Inherit: Same as first input
  X*Y : Outport
  wires:
  X/1 -> Divide2/1
  En/1 -> Divide5/2
  Divide2/1 -> Divide5/1
  Divide5/1 -> X*Y/1
  Y/1 -> Divide2/2

== system EV/SM_Master/Iq_M/Subsystem ==
  X : Inport
  Y : Inport  Port=2
  En : Inport  Port=3
  Divide2 : Product  Inputs=**  OutDataTypeStr=Inherit: Same as first input
  Divide5 : Product  Inputs=**  OutDataTypeStr=Inherit: Same as first input
  X*Y : Outport
  wires:
  X/1 -> Divide2/1
  En/1 -> Divide5/2
  Divide2/1 -> Divide5/1
  Divide5/1 -> X*Y/1
  Y/1 -> Divide2/2

== system EV/SM_Master/Iq_M/Subsystem1 ==
  X : Inport
  Y : Inport  Port=2
  En : Inport  Port=3
  Divide2 : Product  Inputs=**  OutDataTypeStr=Inherit: Same as first input
  Divide5 : Product  Inputs=**  OutDataTypeStr=Inherit: Same as first input
  X*Y : Outport
  wires:
  X/1 -> Divide2/1
  En/1 -> Divide5/2
  Divide2/1 -> Divide5/1
  Divide5/1 -> X*Y/1
  Y/1 -> Divide2/2

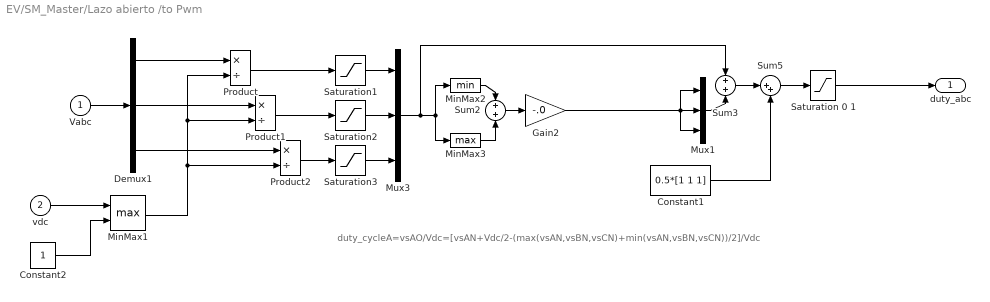
== system EV/SM_Master/Lazo abierto /to Pwm ==
  note: duty_cycleA=vsAO/Vdc=[vsAN+Vdc/2-(max(vsAN,vsBN,vsCN)+min(vsAN,vsBN,vsCN))/2]/Vdc
  Vabc : Inport
  vdc : Inport  Port=2
  Constant1 : Constant  Value=0.5*[1 1 1]
  Constant2 : Constant
  Demux1 : Demux  Outputs=3
  Gain2 : Gain  Gain=-.0  SaturateOnIntegerOverflow=on  OutDataTypeStr=Inherit: Same as input  ParamDataTypeStr=Inherit: Same as input
  MinMax1 : MinMax  Function=max  Inputs=2  InputSameDT=on  SaturateOnIntegerOverflow=on
  MinMax2 : MinMax  InputSameDT=on  SaturateOnIntegerOverflow=on
  MinMax3 : MinMax  Function=max  InputSameDT=on  SaturateOnIntegerOverflow=on
  Mux1 : Mux  Inputs=3
  Mux3 : Mux  Inputs=3
  Product : Product  Inputs=*/  SaturateOnIntegerOverflow=on  OutDataTypeStr=Inherit: Same as first input
  Product1 : Product  Inputs=*/  SaturateOnIntegerOverflow=on  OutDataTypeStr=Inherit: Same as first input
  Product2 : Product  Inputs=*/  SaturateOnIntegerOverflow=on  OutDataTypeStr=Inherit: Same as first input
  Saturation 0 1 : Saturate  UpperLimit=0.98  LowerLimit=0.02
  Saturation1 : Saturate  UpperLimit=1/sqrt(3)  LowerLimit=-1/sqrt(3)
  Saturation2 : Saturate  UpperLimit=1/sqrt(3)  LowerLimit=-1/sqrt(3)
  Saturation3 : Saturate  UpperLimit=1/sqrt(3)  LowerLimit=-1/sqrt(3)
  Sum2 : Sum  InputSameDT=on  SaturateOnIntegerOverflow=on  OutDataTypeStr=Inherit: Same as first input
  Sum3 : Sum  InputSameDT=on  SaturateOnIntegerOverflow=on  OutDataTypeStr=Inherit: Same as first input
  Sum5 : Sum  Inputs=|++  InputSameDT=on  SaturateOnIntegerOverflow=on  OutDataTypeStr=Inherit: Same as first input
  duty_abc : Outport
  wires:
  Sum5/1 -> Saturation 0 1/1
  Mux3/1 -> MinMax3/1, MinMax2/1, Sum3/1
  MinMax3/1 -> Sum2/2
  MinMax2/1 -> Sum2/1
  Sum2/1 -> Gain2/1
  Gain2/1 -> Mux1/2, Mux1/3, Mux1/1
  Sum3/1 -> Sum5/1
  Constant1/1 -> Sum5/2
  Demux1/3 -> Product2/1
  Demux1/1 -> Product/1
  Saturation1/1 -> Mux3/1
  Saturation2/1 -> Mux3/2
  Saturation3/1 -> Mux3/3
  Product/1 -> Saturation1/1
  Product1/1 -> Saturation2/1
  Demux1/2 -> Product1/1
  Product2/1 -> Saturation3/1
  Saturation 0 1/1 -> duty_abc/1
  Mux1/1 -> Sum3/2
  vdc/1 -> MinMax1/1
  MinMax1/1 -> Product2/2, Product1/2, Product/2
  Constant2/1 -> MinMax1/2
  Vabc/1 -> Demux1/1

== system EV/SM_Master/Power Calculator1/Clarke Transformation1 ==
  v-abc : Inport
  Clarke to Beta : Fcn  Expr=0*u[1]+sqrt(1/2)*u[2]-sqrt(1/2)*u[3]
  Clarke to alpha : Fcn  Expr=sqrt(2/3)*u[1]-sqrt(1/6)*u[2]-sqrt(1/6)*u[3]
  v-alpha : Outport
  v-beta : Outport  Port=2
  wires:
  Clarke to Beta/1 -> v-beta/1
  Clarke to alpha/1 -> v-alpha/1
  v-abc/1 -> Clarke to Beta/1, Clarke to alpha/1

== system EV/SM_Master/Power Calculator1/Clarke Transformation2 ==
  v-abc : Inport
  Clarke to Beta : Fcn  Expr=0*u[1]+sqrt(1/2)*u[2]-sqrt(1/2)*u[3]
  Clarke to alpha : Fcn  Expr=sqrt(2/3)*u[1]-sqrt(1/6)*u[2]-sqrt(1/6)*u[3]
  v-alpha : Outport
  v-beta : Outport  Port=2
  wires:
  v-abc/1 -> Clarke to alpha/1, Clarke to Beta/1
  Clarke to alpha/1 -> v-alpha/1
  Clarke to Beta/1 -> v-beta/1

== system EV/SM_Master/Power Calculator1/Filter 1st order 0.7Hz1 ==
  Input : Inport
  Delay11 : Delay  DelayLength=1  InitialCondition=0
  SumA21 : Sum  Inputs=|+-  RndMeth=Nearest  SaturateOnIntegerOverflow=on  OutDataTypeStr=Inherit: Same as first input
  SumB21 : Sum  Inputs=|++  RndMeth=Nearest  SaturateOnIntegerOverflow=on  OutDataTypeStr=Inherit: Same as first input
  a(2)(1) : Gain  Gain=-0.99956027372226808  ParamDataTypeStr=float('double')  RndMeth=Nearest  SaturateOnIntegerOverflow=on  OutDataTypeStr=Inherit: Same as input
  s(1) : Gain  Gain=0.00021986313886602718  ParamDataTypeStr=float('double')  RndMeth=Nearest  SaturateOnIntegerOverflow=on  OutDataTypeStr=Inherit: Same as input
  Output : Outport
  wires:
  Delay11/1 -> SumB21/2, a(2)(1)/1
  a(2)(1)/1 -> SumA21/2
  SumB21/1 -> Output/1
  SumA21/1 -> Delay11/1, SumB21/1
  s(1)/1 -> SumA21/1
  Input/1 -> s(1)/1

== system EV/SM_Master/Power Calculator1/Filter 1st order 0.7Hz2 ==
  Input : Inport
  Delay11 : Delay  DelayLength=1  InitialCondition=0
  SumA21 : Sum  Inputs=|+-  RndMeth=Nearest  SaturateOnIntegerOverflow=on  OutDataTypeStr=Inherit: Same as first input
  SumB21 : Sum  Inputs=|++  RndMeth=Nearest  SaturateOnIntegerOverflow=on  OutDataTypeStr=Inherit: Same as first input
  a(2)(1) : Gain  Gain=-0.99956027372226808  ParamDataTypeStr=float('double')  RndMeth=Nearest  SaturateOnIntegerOverflow=on  OutDataTypeStr=Inherit: Same as input
  s(1) : Gain  Gain=0.00021986313886602718  ParamDataTypeStr=float('double')  RndMeth=Nearest  SaturateOnIntegerOverflow=on  OutDataTypeStr=Inherit: Same as input
  Output : Outport
  wires:
  Input/1 -> s(1)/1
  s(1)/1 -> SumA21/1
  SumA21/1 -> SumB21/1, Delay11/1
  SumB21/1 -> Output/1
  a(2)(1)/1 -> SumA21/2
  Delay11/1 -> a(2)(1)/1, SumB21/2

== system EV/SM_Master/Subsystem2/Gen Rampa ==
  Fase : Inport
  Frec : Inport  Port=2
  En : Inport  Port=3
  Add1 : Sum
  Compare To Constant1 : simulink/Logic and Bit Operations/Compare To Constant  relop=>=  const=2*pi  OutDataTypeStr=boolean
  Gain : Gain  Gain=2*pi
  Gain6 : Gain  Gain=pi/180
  Integrator : Integrator  ExternalReset=rising
  Product : Product
  Unit Delay2 : UnitDelay  SampleTime=Ts  HasFrameUpgradeWarning=on
  "wt " : Outport
  wires:
  Unit Delay2/1 -> Integrator/2
  Add1/1 -> "wt "/1
  En/1 -> Product/2
  Gain6/1 -> Add1/1
  Compare To Constant1/1 -> Unit Delay2/1
  Fase/1 -> Gain6/1
  Gain/1 -> Product/1
  Product/1 -> Integrator/1
  Integrator/1 -> Add1/2, Compare To Constant1/1
  Frec/1 -> Gain/1

== system EV/SM_Master/Vd_M/Subsystem ==
  X : Inport
  Y : Inport  Port=2
  En : Inport  Port=3
  Divide2 : Product  Inputs=**  OutDataTypeStr=Inherit: Same as first input
  Divide5 : Product  Inputs=**  OutDataTypeStr=Inherit: Same as first input
  X*Y : Outport
  wires:
  X/1 -> Divide2/1
  En/1 -> Divide5/2
  Divide2/1 -> Divide5/1
  Divide5/1 -> X*Y/1
  Y/1 -> Divide2/2

== system EV/SM_Master/Vd_M/Subsystem1 ==
  X : Inport
  Y : Inport  Port=2
  En : Inport  Port=3
  Divide2 : Product  Inputs=**  OutDataTypeStr=Inherit: Same as first input
  Divide5 : Product  Inputs=**  OutDataTypeStr=Inherit: Same as first input
  X*Y : Outport
  wires:
  X/1 -> Divide2/1
  En/1 -> Divide5/2
  Divide2/1 -> Divide5/1
  Divide5/1 -> X*Y/1
  Y/1 -> Divide2/2

== system EV/SM_Master/Vd_M1/Subsystem ==
  X : Inport
  Y : Inport  Port=2
  En : Inport  Port=3
  Divide2 : Product  Inputs=**  OutDataTypeStr=Inherit: Same as first input
  Divide5 : Product  Inputs=**  OutDataTypeStr=Inherit: Same as first input
  X*Y : Outport
  wires:
  X/1 -> Divide2/1
  En/1 -> Divide5/2
  Divide2/1 -> Divide5/1
  Divide5/1 -> X*Y/1
  Y/1 -> Divide2/2

== system EV/SM_Master/Vd_M1/Subsystem1 ==
  X : Inport
  Y : Inport  Port=2
  En : Inport  Port=3
  Divide2 : Product  Inputs=**  OutDataTypeStr=Inherit: Same as first input
  Divide5 : Product  Inputs=**  OutDataTypeStr=Inherit: Same as first input
  X*Y : Outport
  wires:
  X/1 -> Divide2/1
  En/1 -> Divide5/2
  Divide2/1 -> Divide5/1
  Divide5/1 -> X*Y/1
  Y/1 -> Divide2/2

== system EV/SM_Master/abc//dq_VM/Subsystem2 ==
  alfa : Inport
  beta : Inport  Port=2
  wt : Inport  Port=3
  Fcn : Fcn  Expr=u(1)*cos(u(3))+u(2)*sin(u(3))
  Fcn1 : Fcn  Expr=-u(1)*sin(u(3))+u(2)*cos(u(3))
  Mux : Mux  Inputs=3
  Mux1 : Mux  Inputs=3
  d : Outport
  Q : Outport  Port=2
  wires:
  Fcn/1 -> d/1
  Fcn1/1 -> Q/1
  Mux/1 -> Fcn/1
  alfa/1 -> Mux1/1, Mux/1
  Mux1/1 -> Fcn1/1
  beta/1 -> Mux1/2, Mux/2
  wt/1 -> Mux1/3, Mux/3

== system EV/SM_Master/abc//dq_VM/abc//alfabeta2 ==
  abc : Inport
  Fcn : Fcn  Expr=1*u(1)-0.5*u(2)-0.5*u(3)
  Fcn1 : Fcn  Expr=0*u(1)+(sqrt(3)/2)*u(2)-(sqrt(3)/2)*u(3)
  Gain : Gain  Gain=k
  alfa : Outport
  Beta : Outport  Port=2
  wires:
  Fcn1/1 -> Beta/1
  Fcn/1 -> alfa/1
  abc/1 -> Gain/1
  Gain/1 -> Fcn/1, Fcn1/1

== system EV/SM_Master/abc//dq_VM1/Subsystem2 ==
  alfa : Inport
  beta : Inport  Port=2
  wt : Inport  Port=3
  Fcn : Fcn  Expr=u(1)*cos(u(3))+u(2)*sin(u(3))
  Fcn1 : Fcn  Expr=-u(1)*sin(u(3))+u(2)*cos(u(3))
  Mux : Mux  Inputs=3
  Mux1 : Mux  Inputs=3
  d : Outport
  Q : Outport  Port=2
  wires:
  wt/1 -> Mux/3, Mux1/3
  beta/1 -> Mux/2, Mux1/2
  Mux1/1 -> Fcn1/1
  alfa/1 -> Mux/1, Mux1/1
  Mux/1 -> Fcn/1
  Fcn1/1 -> Q/1
  Fcn/1 -> d/1

== system EV/SM_Master/abc//dq_VM1/abc//alfabeta2 ==
  abc : Inport
  Fcn : Fcn  Expr=1*u(1)-0.5*u(2)-0.5*u(3)
  Fcn1 : Fcn  Expr=0*u(1)+(sqrt(3)/2)*u(2)-(sqrt(3)/2)*u(3)
  Gain : Gain  Gain=k
  alfa : Outport
  Beta : Outport  Port=2
  wires:
  Gain/1 -> Fcn1/1, Fcn/1
  abc/1 -> Gain/1
  Fcn/1 -> alfa/1
  Fcn1/1 -> Beta/1

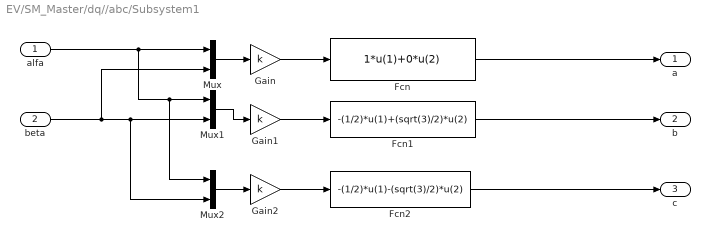
== system EV/SM_Master/dq//abc/Subsystem1 ==
  alfa : Inport
  beta : Inport  Port=2
  Fcn : Fcn  Expr=1*u(1)+0*u(2)
  Fcn1 : Fcn  Expr=-(1/2)*u(1)+(sqrt(3)/2)*u(2)
  Fcn2 : Fcn  Expr=-(1/2)*u(1)-(sqrt(3)/2)*u(2)
  Gain : Gain  Gain=k
  Gain1 : Gain  Gain=k
  Gain2 : Gain  Gain=k
  Mux : Mux  Inputs=2
  Mux1 : Mux  Inputs=2
  Mux2 : Mux  Inputs=2
  a : Outport
  b : Outport  Port=2
  c : Outport  Port=3
  wires:
  alfa/1 -> Mux2/1, Mux1/1, Mux/1
  Fcn2/1 -> c/1
  beta/1 -> Mux/2, Mux2/2, Mux1/2
  Gain1/1 -> Fcn1/1
  Gain2/1 -> Fcn2/1
  Fcn/1 -> a/1
  Mux/1 -> Gain/1
  Gain/1 -> Fcn/1
  Mux1/1 -> Gain1/1
  Mux2/1 -> Gain2/1
  Fcn1/1 -> b/1

== system EV/SM_Master/dq//abc/dq//alfabeta1 ==
  d : Inport
  q : Inport  Port=2
  wt : Inport  Port=3
  Fcn2 : Fcn  Expr=u(1)*cos(u(3))-u(2)*sin(u(3))
  Fcn3 : Fcn  Expr=u(1)*sin(u(3))+u(2)*cos(u(3))
  Mux : Mux  Inputs=3
  Mux1 : Mux  Inputs=3
  alfa : Outport
  beta : Outport  Port=2
  wires:
  Fcn3/1 -> beta/1
  wt/1 -> Mux1/3, Mux/3
  q/1 -> Mux1/2, Mux/2
  Mux/1 -> Fcn2/1
  Fcn2/1 -> alfa/1
  d/1 -> Mux1/1, Mux/1
  Mux1/1 -> Fcn3/1

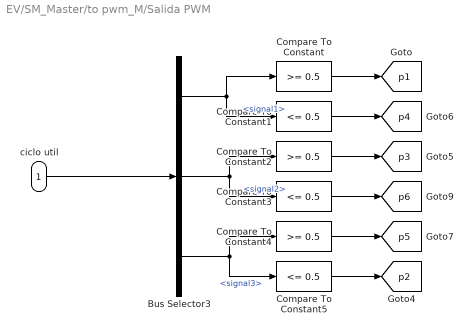
== system EV/SM_Master/to pwm_M/Salida PWM ==
  "ciclo util " : Inport
  Bus Selector3 : BusSelector  OutputSignals=signal1,signal2,signal3
  Compare To Constant : simulink/Logic and Bit Operations/Compare To Constant  relop=>=  const=0.5  OutDataTypeStr=boolean
  Compare To Constant1 : simulink/Logic and Bit Operations/Compare To Constant  relop=<=  const=0.5  OutDataTypeStr=boolean
  Compare To Constant2 : simulink/Logic and Bit Operations/Compare To Constant  relop=>=  const=0.5  OutDataTypeStr=boolean
  Compare To Constant3 : simulink/Logic and Bit Operations/Compare To Constant  relop=<=  const=0.5  OutDataTypeStr=boolean
  Compare To Constant4 : simulink/Logic and Bit Operations/Compare To Constant  relop=>=  const=0.5  OutDataTypeStr=boolean
  Compare To Constant5 : simulink/Logic and Bit Operations/Compare To Constant  relop=<=  const=0.5  OutDataTypeStr=boolean
  tag scope: p1=global, p2=global, p3=global, p4=global, p5=global, p6=global
  wires:
  "ciclo util "/1 -> Bus Selector3/1
  Bus Selector3/1 -> Compare To Constant1/1, Compare To Constant/1  "<signal1>"
  Bus Selector3/2 -> Compare To Constant2/1, Compare To Constant3/1  "<signal2>"
  Bus Selector3/3 -> Compare To Constant5/1, Compare To Constant4/1  "<signal3>"
  Compare To Constant5/1 -> [p2]
  Compare To Constant4/1 -> [p5]
  Compare To Constant3/1 -> [p6]
  Compare To Constant2/1 -> [p3]
  Compare To Constant1/1 -> [p4]
  Compare To Constant/1 -> [p1]

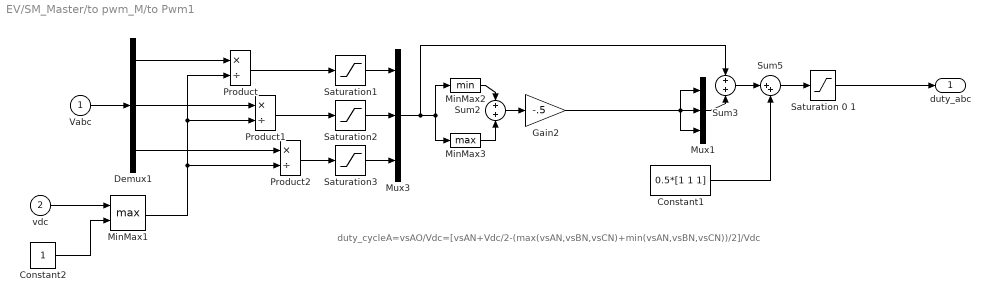
== system EV/SM_Master/to pwm_M/to Pwm1 ==
  note: duty_cycleA=vsAO/Vdc=[vsAN+Vdc/2-(max(vsAN,vsBN,vsCN)+min(vsAN,vsBN,vsCN))/2]/Vdc
  Vabc : Inport
  vdc : Inport  Port=2
  Constant1 : Constant  Value=0.5*[1 1 1]
  Constant2 : Constant
  Demux1 : Demux  Outputs=3
  Gain2 : Gain  Gain=-.5  SaturateOnIntegerOverflow=on  OutDataTypeStr=Inherit: Same as input  ParamDataTypeStr=Inherit: Same as input
  MinMax1 : MinMax  Function=max  Inputs=2  InputSameDT=on  SaturateOnIntegerOverflow=on
  MinMax2 : MinMax  InputSameDT=on  SaturateOnIntegerOverflow=on
  MinMax3 : MinMax  Function=max  InputSameDT=on  SaturateOnIntegerOverflow=on
  Mux1 : Mux  Inputs=3
  Mux3 : Mux  Inputs=3
  Product : Product  Inputs=*/  SaturateOnIntegerOverflow=on  OutDataTypeStr=Inherit: Same as first input
  Product1 : Product  Inputs=*/  SaturateOnIntegerOverflow=on  OutDataTypeStr=Inherit: Same as first input
  Product2 : Product  Inputs=*/  SaturateOnIntegerOverflow=on  OutDataTypeStr=Inherit: Same as first input
  Saturation 0 1 : Saturate  UpperLimit=0.98  LowerLimit=0.02
  Saturation1 : Saturate  UpperLimit=1/sqrt(3)  LowerLimit=-1/sqrt(3)
  Saturation2 : Saturate  UpperLimit=1/sqrt(3)  LowerLimit=-1/sqrt(3)
  Saturation3 : Saturate  UpperLimit=1/sqrt(3)  LowerLimit=-1/sqrt(3)
  Sum2 : Sum  InputSameDT=on  SaturateOnIntegerOverflow=on  OutDataTypeStr=Inherit: Same as first input
  Sum3 : Sum  InputSameDT=on  SaturateOnIntegerOverflow=on  OutDataTypeStr=Inherit: Same as first input
  Sum5 : Sum  Inputs=|++  InputSameDT=on  SaturateOnIntegerOverflow=on  OutDataTypeStr=Inherit: Same as first input
  duty_abc : Outport
  wires:
  Constant2/1 -> MinMax1/2
  MinMax1/1 -> Product/2, Product1/2, Product2/2
  vdc/1 -> MinMax1/1
  Mux1/1 -> Sum3/2
  Vabc/1 -> Demux1/1
  Saturation 0 1/1 -> duty_abc/1
  Product2/1 -> Saturation3/1
  Demux1/2 -> Product1/1
  Product1/1 -> Saturation2/1
  Product/1 -> Saturation1/1
  Saturation3/1 -> Mux3/3
  Saturation2/1 -> Mux3/2
  Saturation1/1 -> Mux3/1
  Demux1/1 -> Product/1
  Demux1/3 -> Product2/1
  Constant1/1 -> Sum5/2
  Sum3/1 -> Sum5/1
  Gain2/1 -> Mux1/1, Mux1/3, Mux1/2
  Sum2/1 -> Gain2/1
  MinMax2/1 -> Sum2/1
  MinMax3/1 -> Sum2/2
  Mux3/1 -> Sum3/1, MinMax2/1, MinMax3/1
  Sum5/1 -> Saturation 0 1/1
